simulink library "nodeDragForce_ul"  (R2020a)
settings: Solver=VariableStepAuto  StartTime=0.0  StopTime=10.0  RelTol=1e-3
settings Model: Creator=mcobb  LastModifiedBy=adabney
settings DataIOCC: ReturnWorkspaceOutputs=off
settings DebuggingCC: ArithmeticOperatorsInVariantConditions=warning
settings SFSimCC: CustomCodeUndefinedFunction=UseInterfaceOnly

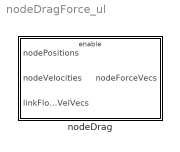
== system nodeDragForce_ul ==
  nodeDrag : Subsystem  mask{flowDensity=0, thrDiam=0, dragCoeff=0}
      mask prompts: flowDensity "Flow Density"; thrDiam "Tether Diameter"; dragCoeff "Drag Coefficient"

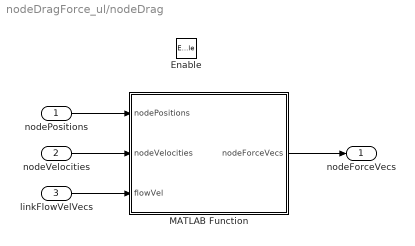
== system nodeDragForce_ul/nodeDrag ==
  nodePositions : Inport
  nodeVelocities : Inport  Port=2
  linkFlowVelVecs : Inport  Port=3
  Enable : EnablePort
  MATLAB Function : MATLAB Function  TreatAsAtomicUnit=on
  nodeForceVecs : Outport  VectorParamsAs1DForOutWhenUnconnected=off
  wires:
  nodeVelocities/1 -> MATLAB Function/2(nodeVelocities)
  MATLAB Function/1(nodeForceVecs) -> nodeForceVecs/1
  nodePositions/1 -> MATLAB Function/1(nodePositions)
  linkFlowVelVecs/1 -> MATLAB Function/3(flowVel)

== matlab function nodeDragForce_ul/nodeDrag/MATLAB Function ==
  data: nodePositions input; nodeForceVecs output; nodeVelocities input; thrDiam parameter; flowDensity parameter; flowVel input; dragCoeff parameter
function nodeForceVecs = fcn(nodePositions,nodeVelocities,thrDiam, flowDensity, flowVel,dragCoeff)

nodeForceVecs = thrNodeDrag(nodePositions,nodeVelocities,thrDiam, flowDensity,flowVel,dragCoeff);

end
